simulink model "External_coordinates_Position_Control"  (R2018b)
settings: Solver=VariableStepAuto  StartTime=0.0  StopTime=15  FixedStep=0.005  RelTol=1e-3
undefined symbols (not defined in the file or in its folder): dt
settings Model: Creator=root  LastModifiedBy=root

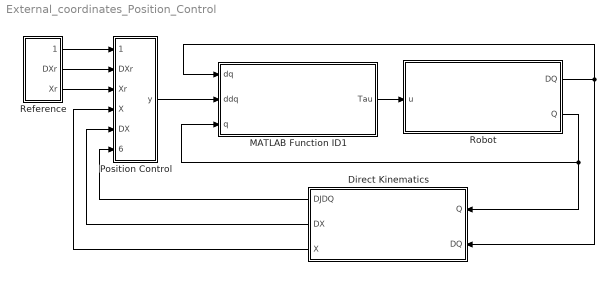
== system External_coordinates_Position_Control ==
  Direct Kinematics : Subsystem
  MATLAB Function ID1 : MATLAB Function  TreatAsAtomicUnit=on
  Position Control : Subsystem
  Reference : Subsystem
  Robot : Subsystem
  wires:
  Position Control/1(y) -> MATLAB Function ID1/2(ddq)
  Robot/2(Q) -> Direct Kinematics/1(Q), MATLAB Function ID1/3(q)
  Reference/2(DXr) -> Position Control/2(DXr)
  Reference/1(DDXr) -> Position Control/1(DDXr)
  Reference/3(Xr) -> Position Control/3(Xr)
  Robot/1(DQ) -> MATLAB Function ID1/1(dq), Direct Kinematics/2(DQ)
  MATLAB Function ID1/1(Tau) -> Robot/1(u)
  Direct Kinematics/1(DJDQ) -> Position Control/6(DJDQ)
  Direct Kinematics/2(DX) -> Position Control/5(DX)
  Direct Kinematics/3(X) -> Position Control/4(X)

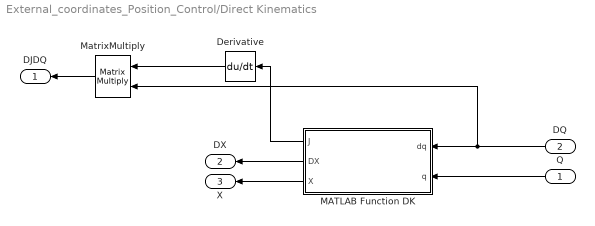
== system External_coordinates_Position_Control/Direct Kinematics ==
  Q : Inport
  DQ : Inport  Port=2
  Derivative : Derivative  CoefficientInTFapproximation=0.001
  MATLAB Function DK : MATLAB Function  TreatAsAtomicUnit=on
  MatrixMultiply : Product  Multiplication=Matrix(*)
  DJDQ : Outport
  DX : Outport  Port=2
  X : Outport  Port=3
  wires:
  MatrixMultiply/1 -> DJDQ/1
  DQ/1 -> MatrixMultiply/2, MATLAB Function DK/1(dq)
  MATLAB Function DK/3(X) -> X/1
  MATLAB Function DK/1(J) -> Derivative/1
  Derivative/1 -> MatrixMultiply/1
  MATLAB Function DK/2(DX) -> DX/1
  Q/1 -> MATLAB Function DK/2(q)

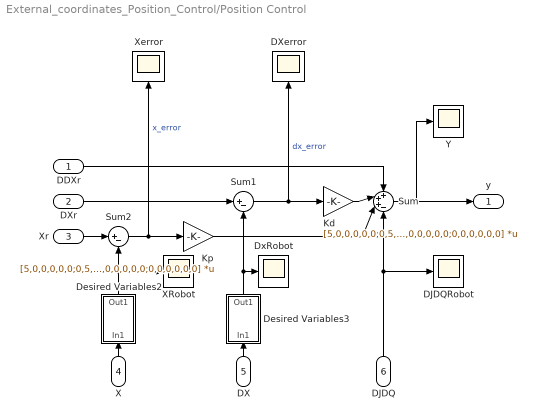
== system External_coordinates_Position_Control/Position Control ==
  DDXr : Inport
  DXr : Inport  Port=2
  Xr : Inport  Port=3
  X : Inport  Port=4
  DX : Inport  Port=5
  DJDQ : Inport  Port=6
  DJDQRobot : Scope
  DXerror : Scope
  Desired Variables2 : Subsystem
  Desired Variables3 : Subsystem
  DxRobot : Scope
  Kd : Gain  Gain=[5,0,0,0,0,0;0,5,0,0,0,0;0,0,5,0,0,0;0,0,0,0,0,0;0,0,0,0,0,0;0,0,0,0,0,0]  Multiplication=Matrix(K*u)
  Kp : Gain  Gain=[5,0,0,0,0,0;0,5,0,0,0,0;0,0,5,0,0,0;0,0,0,0,0,0;0,0,0,0,0,0;0,0,0,0,0,0]  Multiplication=Matrix(K*u)
  Sum : Sum  Inputs=+++-
  Sum1 : Sum  Inputs=|+-
  Sum2 : Sum  Inputs=|+-
  XRobot : Scope
  Xerror : Scope
  Y : Scope
  y : Outport
  wires:
  Kd/1 -> Sum/2
  Kp/1 -> Sum/3
  Sum2/1 -> Xerror/1, Kp/1  "x_error"
  Xr/1 -> Sum2/1
  DXr/1 -> Sum1/1
  Sum1/1 -> DXerror/1, Kd/1  "dx_error"
  Sum/1 -> y/1, Y/1
  DJDQ/1 -> DJDQRobot/1, Sum/4
  DDXr/1 -> Sum/1
  DX/1 -> Desired Variables3/1(In1)
  Desired Variables2/1(Out1) -> Sum2/2, XRobot/1
  Desired Variables3/1(Out1) -> Sum1/2, DxRobot/1
  X/1 -> Desired Variables2/1(In1)

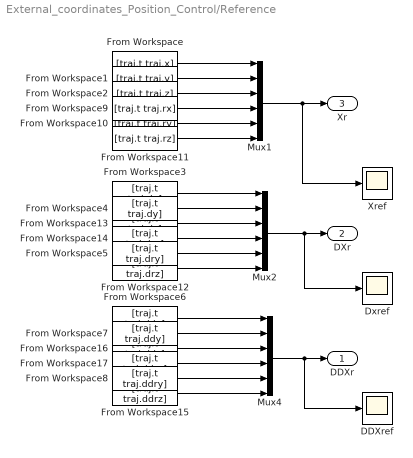
== system External_coordinates_Position_Control/Reference ==
  DDXref : Scope
  Dxref : Scope
  From Workspace : FromWorkspace  VariableName=[traj.t traj.x]  SampleTime=dt  OutputAfterFinalValue=Holding final value
  From Workspace1 : FromWorkspace  VariableName=[traj.t traj.y]  SampleTime=dt  OutputAfterFinalValue=Holding final value
  From Workspace10 : FromWorkspace  VariableName=[traj.t traj.ry]  SampleTime=dt  OutputAfterFinalValue=Holding final value
  From Workspace11 : FromWorkspace  VariableName=[traj.t traj.rz]  SampleTime=dt  OutputAfterFinalValue=Holding final value
  From Workspace12 : FromWorkspace  VariableName=[traj.t traj.drz]  SampleTime=dt  OutputAfterFinalValue=Holding final value
  From Workspace13 : FromWorkspace  VariableName=[traj.t traj.dz]  SampleTime=dt  OutputAfterFinalValue=Holding final value
  From Workspace14 : FromWorkspace  VariableName=[traj.t traj.drx]  SampleTime=dt  OutputAfterFinalValue=Holding final value
  From Workspace15 : FromWorkspace  VariableName=[traj.t traj.ddrz]  SampleTime=dt  OutputAfterFinalValue=Holding final value
  From Workspace16 : FromWorkspace  VariableName=[traj.t traj.ddz]  SampleTime=dt  OutputAfterFinalValue=Holding final value
  From Workspace17 : FromWorkspace  VariableName=[traj.t traj.ddrx]  SampleTime=dt  OutputAfterFinalValue=Holding final value
  From Workspace2 : FromWorkspace  VariableName=[traj.t traj.z]  SampleTime=dt  OutputAfterFinalValue=Holding final value
  From Workspace3 : FromWorkspace  VariableName=[traj.t traj.dx]  SampleTime=dt  OutputAfterFinalValue=Holding final value
  From Workspace4 : FromWorkspace  VariableName=[traj.t traj.dy]  SampleTime=dt  OutputAfterFinalValue=Holding final value
  From Workspace5 : FromWorkspace  VariableName=[traj.t traj.dry]  SampleTime=dt  OutputAfterFinalValue=Holding final value
  From Workspace6 : FromWorkspace  VariableName=[traj.t traj.ddx]  SampleTime=dt  OutputAfterFinalValue=Holding final value
  From Workspace7 : FromWorkspace  VariableName=[traj.t traj.ddy]  SampleTime=dt  OutputAfterFinalValue=Holding final value
  From Workspace8 : FromWorkspace  VariableName=[traj.t traj.ddry]  SampleTime=dt  OutputAfterFinalValue=Holding final value
  From Workspace9 : FromWorkspace  VariableName=[traj.t traj.rx]  SampleTime=dt  OutputAfterFinalValue=Holding final value
  Mux1 : Mux  Inputs=6
  Mux2 : Mux  Inputs=6
  Mux4 : Mux  Inputs=6
  Xref : Scope
  DDXr : Outport
  DXr : Outport  Port=2
  Xr : Outport  Port=3
  wires:
  From Workspace/1 -> Mux1/1
  From Workspace1/1 -> Mux1/2
  From Workspace2/1 -> Mux1/3
  From Workspace11/1 -> Mux1/6
  From Workspace9/1 -> Mux1/4
  From Workspace10/1 -> Mux1/5
  Mux1/1 -> Xref/1, Xr/1
  Mux4/1 -> DDXref/1, DDXr/1
  From Workspace13/1 -> Mux2/3
  From Workspace12/1 -> Mux2/6
  From Workspace3/1 -> Mux2/1
  From Workspace5/1 -> Mux2/5
  From Workspace4/1 -> Mux2/2
  From Workspace14/1 -> Mux2/4
  From Workspace16/1 -> Mux4/3
  From Workspace15/1 -> Mux4/6
  From Workspace6/1 -> Mux4/1
  From Workspace8/1 -> Mux4/5
  From Workspace7/1 -> Mux4/2
  From Workspace17/1 -> Mux4/4
  Mux2/1 -> Dxref/1, DXr/1

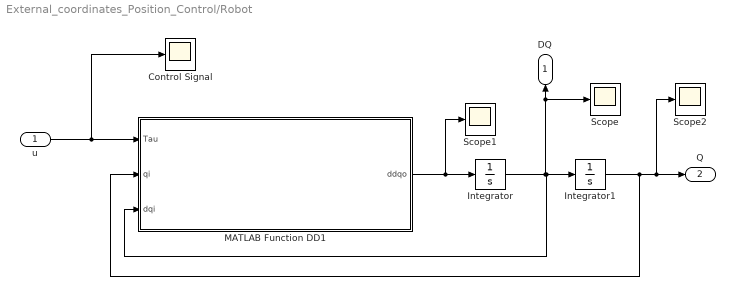
== system External_coordinates_Position_Control/Robot ==
  u : Inport
  Control Signal : Scope
  Integrator : Integrator
  Integrator1 : Integrator  InitialCondition=[0,0,-pi/2,0,-pi/2,0]
  MATLAB Function DD1 : MATLAB Function  TreatAsAtomicUnit=on
  Scope : Scope
  Scope1 : Scope
  Scope2 : Scope
  DQ : Outport
  Q : Outport  Port=2
  wires:
  MATLAB Function DD1/1(ddqo) -> Scope1/1, Integrator/1
  Integrator/1 -> MATLAB Function DD1/3(dqi), Integrator1/1, Scope/1, DQ/1
  Integrator1/1 -> Scope2/1, Q/1, MATLAB Function DD1/2(qi)
  u/1 -> Control Signal/1, MATLAB Function DD1/1(Tau)

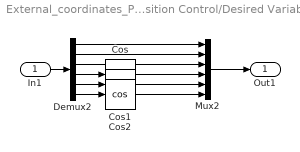
== system External_coordinates_Position_Control/Position Control/Desired Variables2 ==
  In1 : Inport
  Cos : Trigonometry  Operator=cos
  Cos1 : Trigonometry  Operator=cos
  Cos2 : Trigonometry  Operator=cos
  Demux2 : Demux  Outputs=6
  Mux2 : Mux  Inputs=6
  Out1 : Outport
  wires:
  Demux2/3 -> Mux2/3
  Mux2/1 -> Out1/1
  In1/1 -> Demux2/1
  Demux2/4 -> Cos/1
  Demux2/1 -> Mux2/1
  Demux2/6 -> Cos2/1
  Demux2/5 -> Cos1/1
  Demux2/2 -> Mux2/2
  Cos2/1 -> Mux2/6
  Cos1/1 -> Mux2/5
  Cos/1 -> Mux2/4

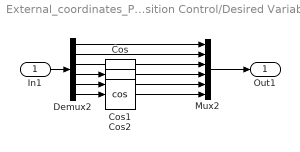
== system External_coordinates_Position_Control/Position Control/Desired Variables3 ==
  In1 : Inport
  Cos : Trigonometry  Operator=cos
  Cos1 : Trigonometry  Operator=cos
  Cos2 : Trigonometry  Operator=cos
  Demux2 : Demux  Outputs=6
  Mux2 : Mux  Inputs=6
  Out1 : Outport
  wires:
  Demux2/3 -> Mux2/3
  Mux2/1 -> Out1/1
  In1/1 -> Demux2/1
  Demux2/4 -> Cos/1
  Demux2/1 -> Mux2/1
  Demux2/6 -> Cos2/1
  Demux2/5 -> Cos1/1
  Demux2/2 -> Mux2/2
  Cos2/1 -> Mux2/6
  Cos1/1 -> Mux2/5
  Cos/1 -> Mux2/4

== matlab function External_coordinates_Position_Control/Direct Kinematics/MATLAB Function DK ==
  data: J output; dq input; q input; DX output; X output
function [J,DX,X]   = Direct_Kinematics(dq,q)
    J = zeros(6,6);
    X = zeros(6,1);
    DX = zeros(6,1);
    DJDQ = zeros(6,1);
    coder.extrinsic('JacobianUR3');
    coder.extrinsic('Direct_Kinematics');
    J = JacobianUR3(q);
    X = Direct_Kinematics(q);
    DX = J*dq;
end

== matlab function External_coordinates_Position_Control/Robot/MATLAB Function DD1 ==
  data: Tau input; ddqo output; qi input; dqi input
function ddqo = DirectDynamics(Tau,qi,dqi)
    ddqo = zeros(6,1);
    coder.extrinsic('SolveSyms');
    c = zeros(6,1);
    m = zeros(6,6);
    g = zeros(6,1);
    [m,g,c] = SolveSyms(qi,dqi);
    ddqo = m\(Tau-c-g);
end

== matlab function External_coordinates_Position_Control/MATLAB Function ID1 ==
  data: dq input; ddq input; q input; Tau output
function Tau   = Inverse_Dynamics(dq,ddq,q)
    coder.extrinsic('SolveSyms');
    coder.extrinsic('JacobianUR3');
    Tau = zeros(6,1);
    c = zeros(6,1);
    m = zeros(6,6);
    g = zeros(6,1);
    J = zeros(6);
    [m,g,c] = SolveSyms(q,dq);
    J = JacobianUR3(q);
    ddq = J\ddq;
    Tau = (m*ddq + c + g);
end
